simulink model "main_control_scheme"  (R2023b)
settings: Solver=VariableStepAuto  StartTime=0.0  StopTime=10  RelTol=1e-3
libraries: instrumentlib x2
settings Model: Creator=pc  LastModifiedBy=pc

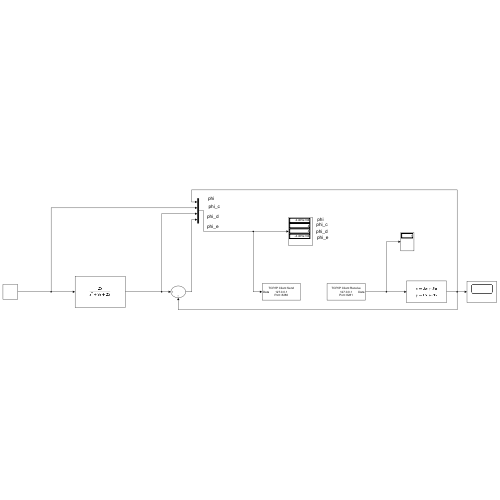
[thumbnail: Simulink's stored preview of the top-level diagram]
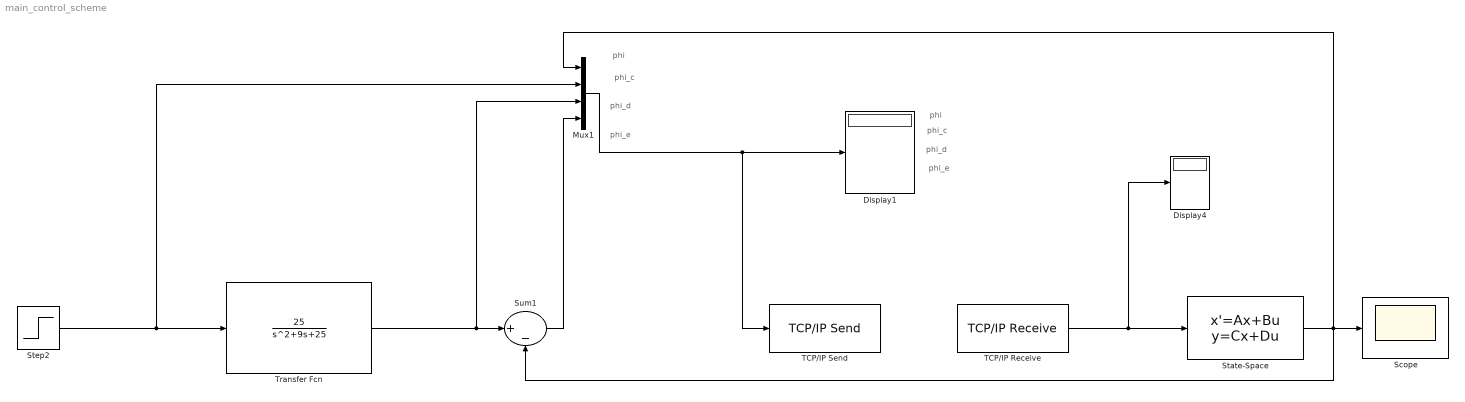
== system main_control_scheme ==
  note: phi_e
  note: phi
  note: phi_c
  note: phi_d
  note: phi_c
  note: phi_d
  note: phi_e
  note: phi
  Display1 : Display
  Display4 : Display
      settings: Decimation=3
  Mux1 : Mux
  Scope : Scope
  State-Space : StateSpace  D=0  InitialCondition=1  ContinuousStateAttributes='Controlled_Object'
  Step2 : Step  Time=0  Before=4.0  After=4.0  SampleTime=0
  Sum1 : Sum  Inputs=|+-
  TCP/IP Receive : instrumentlib/TCP//IP Receive  Host=127.0.0.1  Port=8281  DataSize=[1]  DataType=double  ASCIIFormatting=%f  Terminator=LF  CustomTerminator=10  ByteOrder=big-endian  EnableBlockingMode=on  Timeout=10  SampleTime=0.01  SimulateUsing=Interpreted execution
  TCP/IP Send : instrumentlib/TCP//IP Send  Host=127.0.0.1  Port=8280  ByteOrder=big-endian  EnableBlockingMode=on  Timeout=10  TransferDelay=on  SimulateUsing=Interpreted execution
  Transfer Fcn : TransferFcn  Numerator=[25]  Denominator=[1 9 25]  ContinuousStateAttributes='Reference_Model'
  wires:
  Step2/1 -> Mux1/2, Transfer Fcn/1
  Transfer Fcn/1 -> Sum1/1, Mux1/3
  State-Space/1 -> Mux1/1, Sum1/2, Scope/1
  TCP/IP Receive/1 -> Display4/1, State-Space/1
  Mux1/1 -> TCP/IP Send/1, Display1/1
  Sum1/1 -> Mux1/4
